simulink model "AtherEnergyAretimusRuralDriveCycleInputs"  (R2018a)
settings: Solver=FixedStepAuto  StartTime=0.0  StopTime=82  FixedStep=0.0001  RelTol=1e-3
values from neighbouring files (symbols this model uses):
  A = 1.8585    [Ather_Energy_450.m]
  cd = 0.15    [Ather_Energy_450.m]
  crf = 0.015    [Ather_Energy_450.m]
  GR = 15    [Ather_Energy_450.m]
  GVM = M+Md    (= 400)    [Ather_Energy_450.m]
  GVW = GVM*g    (= 3924)    [Ather_Energy_450.m]
  rho = 1.2250    (= 1.225)    [Ather_Energy_450.m]
  Rw = 0.2286    [Ather_Energy_450.m]
  Teff = 0.85    [Ather_Energy_450.m]
settings Model: Creator=VAISHNAV  LastModifiedBy=VAISHNAV

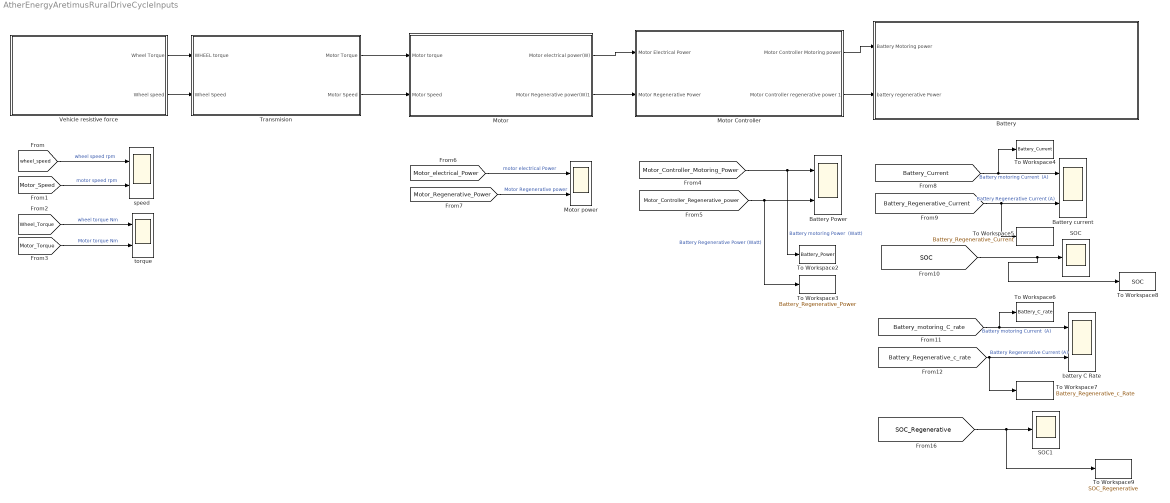
== system AtherEnergyAretimusRuralDriveCycleInputs ==
  Battery : Subsystem
  Battery Power : Scope  NumInputPorts=2
  "Battery current " : Scope  NumInputPorts=2
  Motor : Subsystem
  Motor Controller : Subsystem
  Motor power : Scope  NumInputPorts=2
  SOC : Scope
  SOC1 : Scope
  To Workspace2 : ToWorkspace  VariableName=Battery_Power  SaveFormat=Timeseries  SampleTime=-1
  To Workspace3 : ToWorkspace  VariableName=Battery_Regenerative_Power  SaveFormat=Timeseries  SampleTime=-1
  To Workspace4 : ToWorkspace  VariableName=Battery_Current  SaveFormat=Timeseries  SampleTime=-1
  To Workspace5 : ToWorkspace  VariableName=Battery_Regenerative_Current  SaveFormat=Timeseries  SampleTime=-1
  To Workspace6 : ToWorkspace  VariableName=Battery_C_rate  SaveFormat=Timeseries  SampleTime=-1
  To Workspace7 : ToWorkspace  VariableName=Battery_Regenerative_c_Rate  SaveFormat=Timeseries  SampleTime=-1
  To Workspace8 : ToWorkspace  VariableName=SOC  SaveFormat=Timeseries  SampleTime=-1
  To Workspace9 : ToWorkspace  VariableName=SOC_Regenerative  SaveFormat=Timeseries  SampleTime=-1
  Transmision : Subsystem
  Vehicle resistive force : Subsystem
  battery C Rate : Scope  NumInputPorts=2
  speed : Scope  NumInputPorts=2
  torque : Scope  NumInputPorts=2
  wires:
  Vehicle resistive force/1(Wheel Torque) -> Transmision/1(WHEEL torque)
  Vehicle resistive force/2(Wheel speed) -> Transmision/2(Wheel Speed)
  [Motor_Torque] -> torque/2  "Motor torque Nm"
  [Motor_Speed] -> speed/2  "motor speed rpm"
  [wheel_speed] -> speed/1  "wheel speed rpm"
  [Wheel_Torque] -> torque/1  "wheel torque Nm"
  [Motor_electrical_Power] -> Motor power/1  "motor electrical Power"
  [Motor_Regenerative_Power] -> Motor power/2  "Motor Regenerative power"
  Transmision/1(Motor Torque) -> Motor/1(Motor torque)
  Transmision/2(Motor Speed) -> Motor/2(Motor Speed)
  [Motor_Controller_Motoring_Power] -> To Workspace2/1, Battery Power/1  "Battery motoring Power  (Watt)"
  [Motor_Controller_Regenerative_power] -> To Workspace3/1, Battery Power/2  "Battery Regenerative Power (Watt)"
  [SOC_Regenerative] -> To Workspace9/1, SOC1/1
  [Battery_Regenerative_Current] -> To Workspace5/1, "Battery current "/2  "Battery Regenerative Current (A)"
  [Battery_motoring_C_rate] -> To Workspace6/1, battery C Rate/1  "Battery motoring Current  (A)"
  [Battery_Current] -> To Workspace4/1, "Battery current "/1  "Battery motoring Current  (A)"
  [Battery_Regenerative_c_rate] -> To Workspace7/1, battery C Rate/2  "Battery Regenerative Current (A)"
  [SOC] -> To Workspace8/1, SOC/1
  Motor/1(Motor electrical power(W)) -> Motor Controller/1(Motor Electrical Power)
  Motor/2(Motor Regenerative power(W)1) -> Motor Controller/2(Motor Regenerative Power)
  Motor Controller/1("Motor Controller Motoring power ") -> Battery/1(Battery Motoring power)
  Motor Controller/2(Motor Controller regenerative power 1) -> Battery/2(battery regenerative Power)

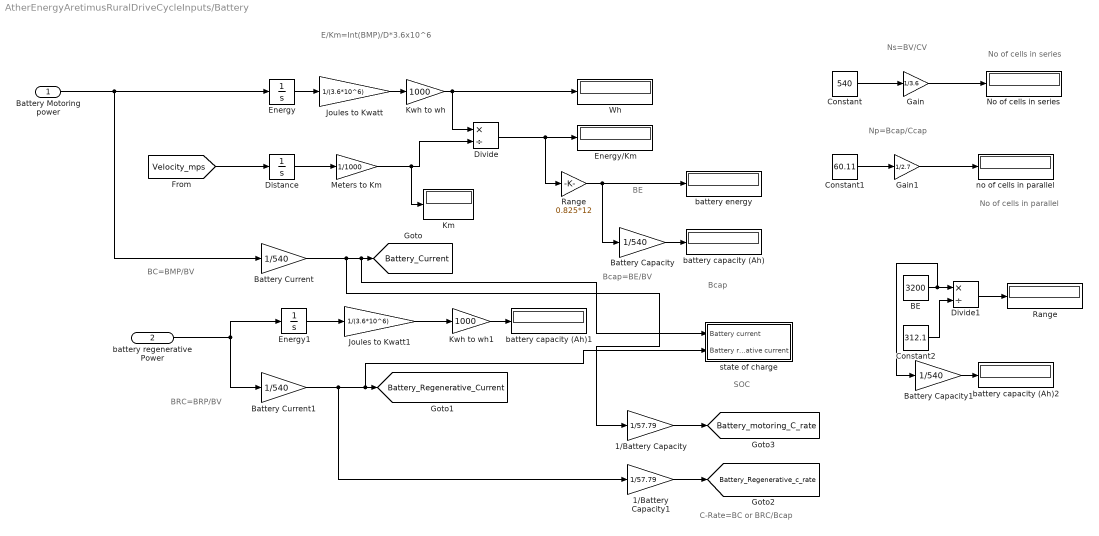
== system AtherEnergyAretimusRuralDriveCycleInputs/Battery ==
  note: Np=Bcap/Ccap
  note: BRC=BRP/BV
  note: No of cells in parallel
  note: Bcap=BE/BV
  note: C-Rate=BC or BRC/Bcap
  note: Bcap
  note: No of cells in series
  note: Ns=BV/CV
  note: BC=BMP/BV
  note: BE
  note: E/Km=Int(BMP)/D*3.6x10^6
  note: SOC
  Battery Motoring power : Inport
  battery regenerative Power : Inport  Port=2
  1/Battery Capacity : Gain  Gain=1/57.79
  1/Battery Capacity1 : Gain  Gain=1/57.79
  BE : Constant  Value=3200
  Battery Capacity : Gain  Gain=1/540
  Battery Capacity1 : Gain  Gain=1/540
  Battery Current : Gain  Gain=1/540
  Battery Current1 : Gain  Gain=1/540
  Constant : Constant  Value=540
  Constant1 : Constant  Value=60.11
  Constant2 : Constant  Value=312.1
  Distance : Integrator
  Divide : Product  Inputs=*/
  Divide1 : Product  Inputs=*/
  Energy : Integrator
  Energy/Km : Display
  Energy1 : Integrator
  Gain : Gain  Gain=1/3.6
  Gain1 : Gain  Gain=1/2.7
  Joules to Kwatt : Gain  Gain=1/(3.6*10^6)
  Joules to Kwatt1 : Gain  Gain=1/(3.6*10^6)
  Km : Display
  Kwh to wh : Gain  Gain=1000
  Kwh to wh1 : Gain  Gain=1000
  Meters to Km : Gain  Gain=1/1000
  No of cells in series : Display
  Range : Gain  Gain=0.825*12
  "Range " : Display
  Wh : Display
  battery capacity (Ah) : Display
  battery capacity (Ah)1 : Display
  battery capacity (Ah)2 : Display
  battery energy : Display
  no of cells in parallel : Display
  state of charge : Subsystem
  tag scope: Battery_Current=global, Battery_Regenerative_Current=global, Battery_Regenerative_c_rate=global, Battery_motoring_C_rate=global
  wires:
  Kwh to wh/1 -> Wh/1, Divide/1
  Constant2/1 -> Divide1/2
  Battery Capacity1/1 -> battery capacity (Ah)2/1
  BE/1 -> Battery Capacity1/1, Divide1/1
  Joules to Kwatt/1 -> Kwh to wh/1
  Constant1/1 -> Gain1/1
  Gain/1 -> No of cells in series/1
  battery regenerative Power/1 -> Energy1/1, Battery Current1/1
  Range/1 -> Battery Capacity/1, battery energy/1
  Kwh to wh1/1 -> battery capacity (Ah)1/1
  Energy1/1 -> Joules to Kwatt1/1
  Gain1/1 -> no of cells in parallel/1
  Constant/1 -> Gain/1
  Distance/1 -> Meters to Km/1
  Battery Current/1 -> 1/Battery Capacity/1, state of charge/1(Battery current), [Battery_Current]
  1/Battery Capacity1/1 -> [Battery_Regenerative_c_rate]
  Joules to Kwatt1/1 -> Kwh to wh1/1
  1/Battery Capacity/1 -> [Battery_motoring_C_rate]
  Divide/1 -> Range/1, Energy/Km/1
  Energy/1 -> Joules to Kwatt/1
  [Velocity_mps] -> Distance/1
  Battery Current1/1 -> 1/Battery Capacity1/1, state of charge/2("Battery regenerative current "), [Battery_Regenerative_Current]
  Divide1/1 -> "Range "/1
  Battery Motoring power/1 -> Energy/1, Battery Current/1
  Meters to Km/1 -> Km/1, Divide/2
  Battery Capacity/1 -> battery capacity (Ah)/1

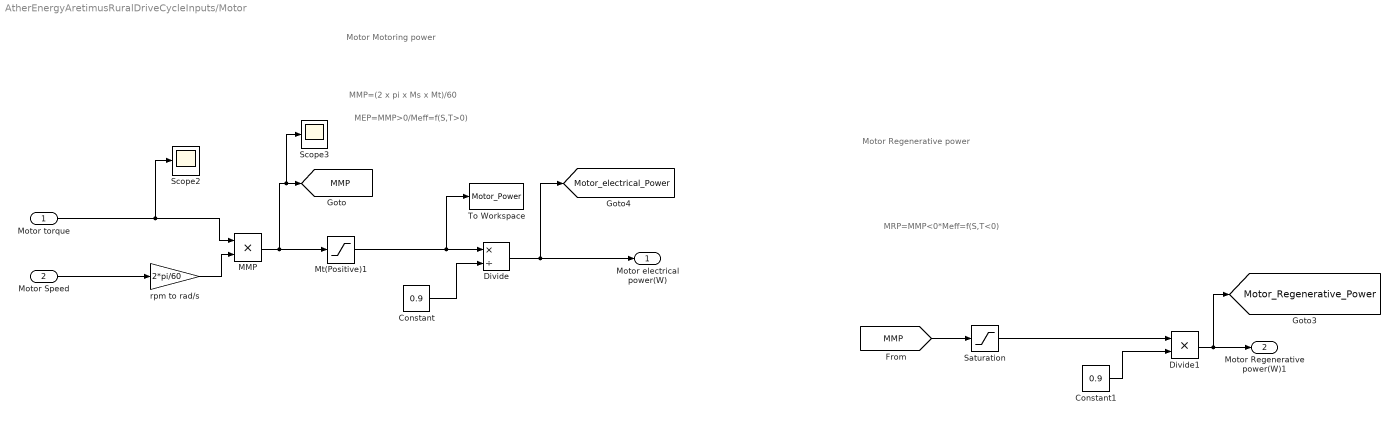
== system AtherEnergyAretimusRuralDriveCycleInputs/Motor ==
  note: MEP=MMP>0/Meff=f(S,T>0)
  note: Motor Motoring power
  note: MMP=(2 x pi x Ms x Mt)/60
  note: MRP=MMP<0*Meff=f(S,T<0)
  note: Motor Regenerative power
  Motor torque : Inport
  Motor Speed : Inport  Port=2
  Constant : Constant  Value=0.9
  Constant1 : Constant  Value=0.9
  Divide : Product  Inputs=*/
  Divide1 : Product  Inputs=**
  MMP : Product
  Mt(Positive)1 : Saturate  UpperLimit=inf  LowerLimit=0
  Saturation : Saturate  UpperLimit=0  LowerLimit=-inf
  Scope2 : Scope
  Scope3 : Scope
  To Workspace : ToWorkspace  VariableName=Motor_Power  SaveFormat=Timeseries  SampleTime=-1
  rpm to rad/s : Gain  Gain=2*pi/60
  Motor electrical power(W) : Outport
  Motor Regenerative power(W)1 : Outport  Port=2
  tag scope: MMP=global, Motor_Regenerative_Power=global, Motor_electrical_Power=global
  wires:
  Constant/1 -> Divide/2
  Motor torque/1 -> Scope2/1, MMP/1
  rpm to rad/s/1 -> MMP/2
  Divide/1 -> [Motor_electrical_Power], Motor electrical power(W)/1
  MMP/1 -> Scope3/1, [MMP], Mt(Positive)1/1
  Motor Speed/1 -> rpm to rad/s/1
  Mt(Positive)1/1 -> To Workspace/1, Divide/1
  Divide1/1 -> [Motor_Regenerative_Power], Motor Regenerative power(W)1/1
  Constant1/1 -> Divide1/2
  Saturation/1 -> Divide1/1
  [MMP] -> Saturation/1

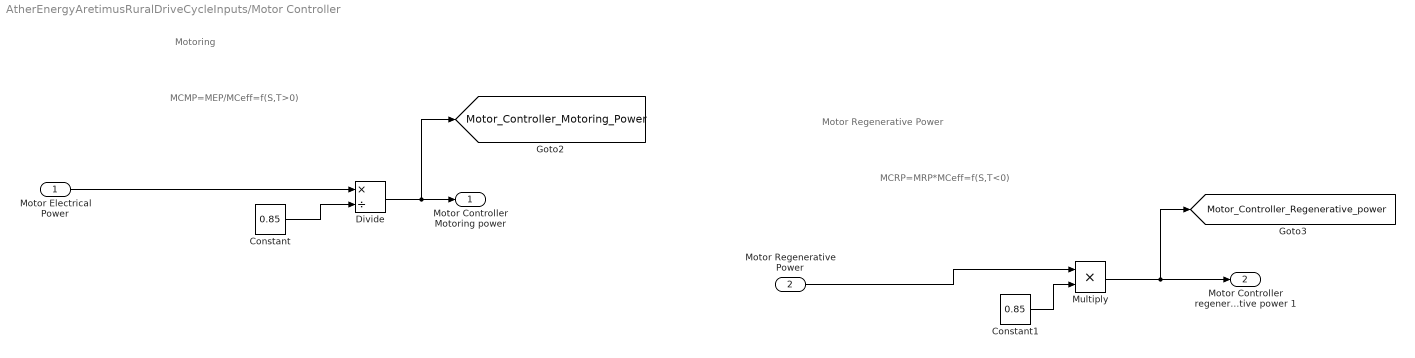
== system AtherEnergyAretimusRuralDriveCycleInputs/Motor Controller ==
  note: Motoring
  note: MCMP=MEP/MCeff=f(S,T>0)
  note: MCRP=MRP*MCeff=f(S,T<0)
  note: Motor Regenerative Power
  Motor Electrical Power : Inport
  Motor Regenerative Power : Inport  Port=2
  Constant : Constant  Value=0.85
  Constant1 : Constant  Value=0.85
  Divide : Product  Inputs=*/
  Multiply : Product
  "Motor Controller Motoring power " : Outport
  Motor Controller regenerative power 1 : Outport  Port=2
  tag scope: Motor_Controller_Motoring_Power=global, Motor_Controller_Regenerative_power=global
  wires:
  Divide/1 -> [Motor_Controller_Motoring_Power], "Motor Controller Motoring power "/1
  Constant/1 -> Divide/2
  Motor Electrical Power/1 -> Divide/1
  Constant1/1 -> Multiply/2
  Motor Regenerative Power/1 -> Multiply/1
  Multiply/1 -> [Motor_Controller_Regenerative_power], Motor Controller regenerative power 1/1

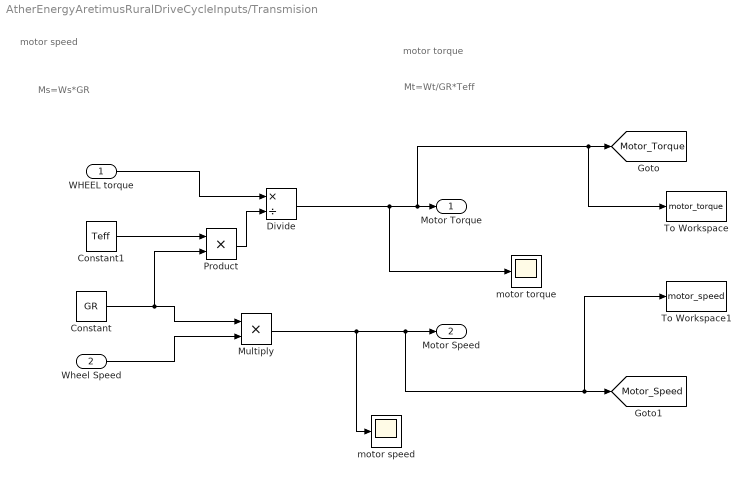
== system AtherEnergyAretimusRuralDriveCycleInputs/Transmision ==
  note: motor torque
  note: Mt=Wt/GR*Teff
  note: Ms=Ws*GR
  note: motor speed
  WHEEL torque : Inport
  Wheel Speed : Inport  Port=2
  Constant : Constant  Value=GR
  Constant1 : Constant  Value=Teff
  Divide : Product  Inputs=*/
  Multiply : Product
  Product : Product
  To Workspace : ToWorkspace  VariableName=motor_torque  SaveFormat=Timeseries  SampleTime=-1
  To Workspace1 : ToWorkspace  VariableName=motor_speed  SaveFormat=Timeseries  SampleTime=-1
  motor speed : Scope
  motor torque : Scope
  Motor Torque : Outport
  Motor Speed : Outport  Port=2
  tag scope: Motor_Speed=global, Motor_Torque=global
  wires:
  Constant1/1 -> Product/1
  Product/1 -> Divide/2
  Divide/1 -> motor torque/1, To Workspace/1, [Motor_Torque], Motor Torque/1
  WHEEL torque/1 -> Divide/1
  Constant/1 -> Product/2, Multiply/1
  Wheel Speed/1 -> Multiply/2
  Multiply/1 -> motor speed/1, To Workspace1/1, [Motor_Speed], Motor Speed/1

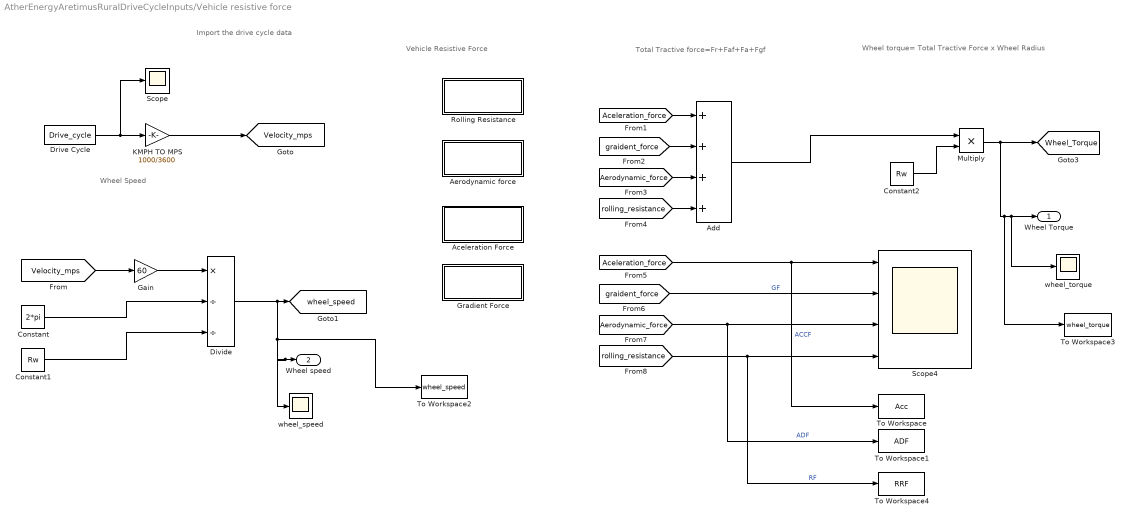
== system AtherEnergyAretimusRuralDriveCycleInputs/Vehicle resistive force ==
  note: Vehicle Resistive Force
  note: Wheel Speed
  note: Wheel torque= Total Tractive Force x Wheel Radius
  note: Import the drive cycle data
  note: Total Tractive force=Fr+Faf+Fa+Fgf
  Aceleration Force : Subsystem
  Add : Sum  Inputs=++++
  Aerodynamic force : Subsystem
  Constant : Constant  Value=2*pi
  Constant1 : Constant  Value=Rw
  Constant2 : Constant  Value=Rw
  Divide : Product  Inputs=*//
  Drive Cycle : FromWorkspace  VariableName=Drive_cycle  SampleTime=0
  Gain : Gain  Gain=60
  Gradient Force : Subsystem
  KMPH TO MPS : Gain  Gain=1000/3600
  Multiply : Product
  Rolling Resistance : Subsystem
  Scope : Scope
  Scope4 : Scope  NumInputPorts=4
  To Workspace : ToWorkspace  VariableName=Acc  SaveFormat=Timeseries  SampleTime=-1
  To Workspace1 : ToWorkspace  VariableName=ADF  SaveFormat=Timeseries  SampleTime=-1
  To Workspace2 : ToWorkspace  VariableName=wheel_speed  SaveFormat=Timeseries  SampleTime=-1
  To Workspace3 : ToWorkspace  VariableName=wheel_torque  SaveFormat=Timeseries  SampleTime=-1
  To Workspace4 : ToWorkspace  VariableName=RRF  SaveFormat=Timeseries  SampleTime=-1
  wheel_speed : Scope
  wheel_torque : Scope
  Wheel Torque : Outport
  Wheel speed : Outport  Port=2
  tag scope: Velocity_mps=global, Wheel_Torque=global, wheel_speed=global
  wires:
  [Velocity_mps] -> Gain/1
  [rolling_resistance] -> To Workspace4/1, Scope4/4  "RF"
  [graident_force] -> Scope4/2  "GF"
  Constant1/1 -> Divide/3
  [Aceleration_force] -> Add/1
  [graident_force] -> Add/2
  [Aerodynamic_force] -> Add/3
  Constant2/1 -> Multiply/2
  Gain/1 -> Divide/1
  Divide/1 -> To Workspace2/1, wheel_speed/1, Wheel speed/1, [wheel_speed]
  Constant/1 -> Divide/2
  KMPH TO MPS/1 -> [Velocity_mps]
  Multiply/1 -> To Workspace3/1, wheel_torque/1, Wheel Torque/1, [Wheel_Torque]
  [rolling_resistance] -> Add/4
  Drive Cycle/1 -> Scope/1, KMPH TO MPS/1
  Add/1 -> Multiply/1
  [Aceleration_force] -> To Workspace/1, Scope4/1  "ACCF"
  [Aerodynamic_force] -> To Workspace1/1, Scope4/3  "ADF"

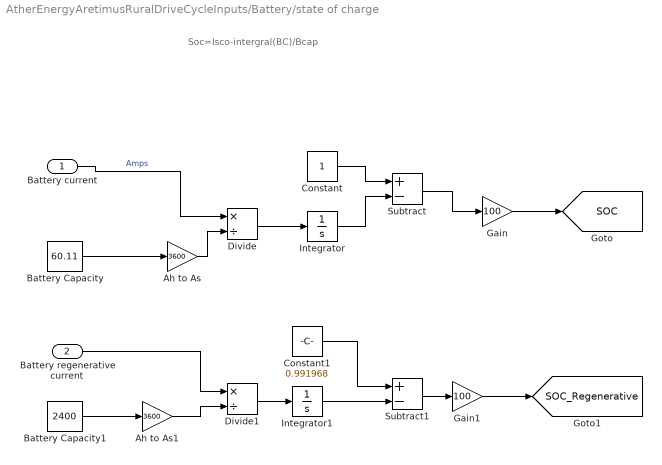
== system AtherEnergyAretimusRuralDriveCycleInputs/Battery/state of charge ==
  note: Soc=Isco-intergral(BC)/Bcap
  Battery current : Inport
  "Battery regenerative current " : Inport  Port=2
  Ah to As : Gain  Gain=3600
  Ah to As1 : Gain  Gain=3600
  Battery Capacity : Constant  Value=60.11
  Battery Capacity1 : Constant  Value=2400
  Constant : Constant
  Constant1 : Constant  Value=0.991968
  Divide : Product  Inputs=*/
  Divide1 : Product  Inputs=*/
  Gain : Gain  Gain=100
  Gain1 : Gain  Gain=100
  Integrator : Integrator
  Integrator1 : Integrator
  Subtract : Sum  Inputs=+-
  Subtract1 : Sum  Inputs=+-
  tag scope: SOC=global, SOC_Regenerative=global
  wires:
  Ah to As/1 -> Divide/2
  Battery Capacity/1 -> Ah to As/1
  Battery current/1 -> Divide/1  "Amps"
  Divide/1 -> Integrator/1
  Gain/1 -> [SOC]
  Integrator/1 -> Subtract/2
  Constant/1 -> Subtract/1
  Subtract/1 -> Gain/1
  Battery Capacity1/1 -> Ah to As1/1
  Ah to As1/1 -> Divide1/2
  "Battery regenerative current "/1 -> Divide1/1
  Divide1/1 -> Integrator1/1
  Integrator1/1 -> Subtract1/2
  Constant1/1 -> Subtract1/1
  Subtract1/1 -> Gain1/1
  Gain1/1 -> [SOC_Regenerative]

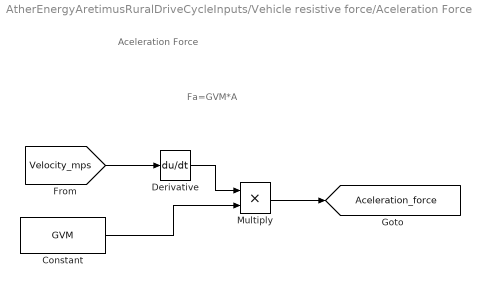
== system AtherEnergyAretimusRuralDriveCycleInputs/Vehicle resistive force/Aceleration Force ==
  note: Fa=GVM*A
  note: Aceleration Force
  Constant : Constant  Value=GVM
  Derivative : Derivative
  Multiply : Product
  tag scope: Aceleration_force=global
  wires:
  Constant/1 -> Multiply/2
  Multiply/1 -> [Aceleration_force]
  [Velocity_mps] -> Derivative/1
  Derivative/1 -> Multiply/1

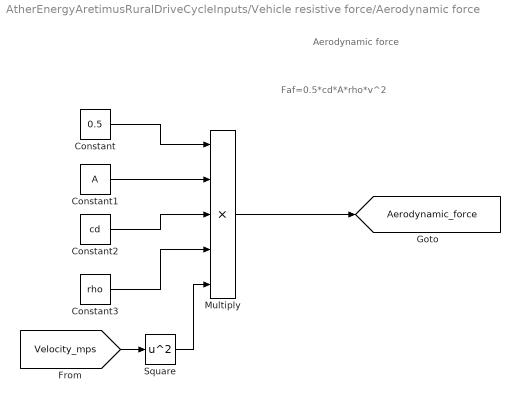
== system AtherEnergyAretimusRuralDriveCycleInputs/Vehicle resistive force/Aerodynamic force ==
  note: Faf=0.5*cd*A*rho*v^2
  note: Aerodynamic force
  Constant : Constant  Value=0.5
  Constant1 : Constant  Value=A
  Constant2 : Constant  Value=cd
  Constant3 : Constant  Value=rho
  Multiply : Product  Inputs=5
  Square : Math  Operator=square  SaturateOnIntegerOverflow=on
  tag scope: Aerodynamic_force=global
  wires:
  Constant/1 -> Multiply/1
  Constant1/1 -> Multiply/2
  Constant2/1 -> Multiply/3
  Constant3/1 -> Multiply/4
  Multiply/1 -> [Aerodynamic_force]
  [Velocity_mps] -> Square/1
  Square/1 -> Multiply/5

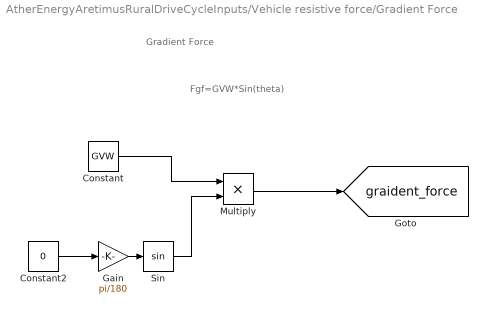
== system AtherEnergyAretimusRuralDriveCycleInputs/Vehicle resistive force/Gradient Force ==
  note: Fgf=GVW*Sin(theta)
  note: Gradient Force
  Constant : Constant  Value=GVW
  Constant2 : Constant  Value=0
  Gain : Gain  Gain=pi/180
  Multiply : Product
  Sin : Trigonometry
  tag scope: graident_force=global
  wires:
  Multiply/1 -> [graident_force]
  Constant/1 -> Multiply/1
  Sin/1 -> Multiply/2
  Gain/1 -> Sin/1
  Constant2/1 -> Gain/1

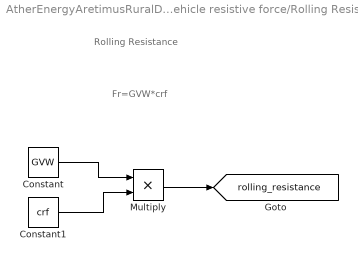
== system AtherEnergyAretimusRuralDriveCycleInputs/Vehicle resistive force/Rolling Resistance ==
  note: Fr=GVW*crf
  note: Rolling Resistance
  Constant : Constant  Value=GVW
  Constant1 : Constant  Value=crf
  Multiply : Product
  tag scope: rolling_resistance=global
  wires:
  Constant/1 -> Multiply/1
  Constant1/1 -> Multiply/2
  Multiply/1 -> [rolling_resistance]
